simulink model "FSFB"  (R2023a)
settings: Solver=VariableStepAuto  StartTime=0.0  StopTime=60  RelTol=1e-8
values from neighbouring files (symbols this model uses):
  e_0 = [0;0;0]    [as5.m]
  eps_0 = [.2; -.5; .3]    [as5.m]
  eps_c = [-.2; -.4; .2]    [as5.m]
  eta_0 = sqrt(1- eps_0'*eps_0)    [as5.m]
  eta_c = sqrt(1- eps_c'*eps_c)    [as5.m]
  I = [1200 0 0; 0 2000 0; 0 0 2800]    [as5.m]
  k_d = I * eye(3) * 2 * zeta * omega_n    [as5.m]
  k_p = I * eye(3) * 2 * omega_n^2    [as5.m]
  omega_0 = [.1; -.05; .05]    [as5.m]
settings Model: Creator=renob  LastModifiedBy=rbrown

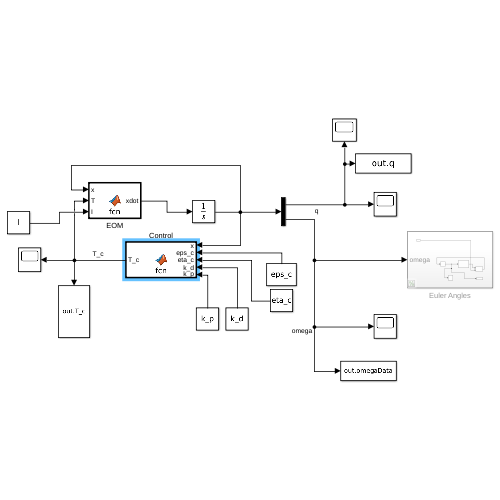
[thumbnail: Simulink's stored preview of the top-level diagram]
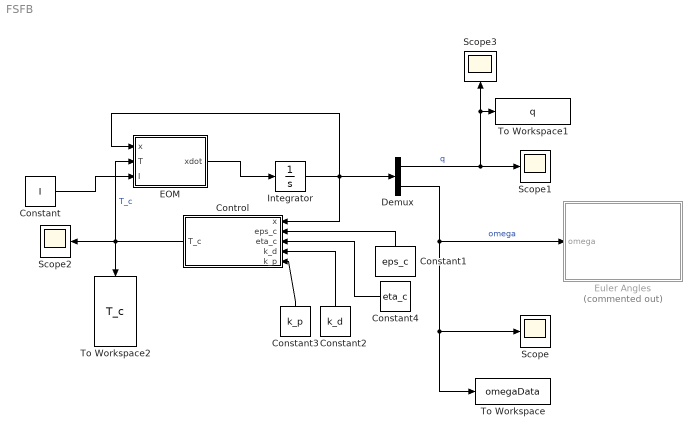
== system FSFB ==
  Constant : Constant  Value=I
  Constant1 : Constant  Value=eps_c
  Constant2 : Constant  Value=k_d
  Constant3 : Constant  Value=k_p  VectorParams1D=off
  Constant4 : Constant  Value=eta_c
  Control : MATLAB Function  TreatAsAtomicUnit=on
  Demux : Demux  Outputs=[-1 3]
  EOM : MATLAB Function  TreatAsAtomicUnit=on
  Euler Angles : Subsystem  Commented=on
  Integrator : Integrator  InitialCondition=[eps_0; eta_0; omega_0]
  Scope{,1..3} (4 alike) : Scope
  To Workspace : ToWorkspace  VariableName=omegaData  SampleTime=-1
  To Workspace1 : ToWorkspace  VariableName=q  SampleTime=-1
  To Workspace2 : ToWorkspace  VariableName=T_c  SampleTime=-1
      settings: Save2DSignal=2-D array (concatenate along first dimension)
  wires:
  Demux/2 -> To Workspace/1, Scope/1, Euler Angles/1(omega)  "omega"
  Demux/1 -> Scope1/1, Scope3/1, To Workspace1/1  "q"
  Constant/1 -> EOM/3(I)
  Integrator/1 -> Control/1(x), EOM/1(x), Demux/1
  EOM/1(xdot) -> Integrator/1
  Control/1(T_c) -> To Workspace2/1, Scope2/1, EOM/2(T)  "T_c"
  Constant1/1 -> Control/2(eps_c)
  Constant2/1 -> Control/4(k_d)
  Constant3/1 -> Control/5(k_p)
  Constant4/1 -> Control/3(eta_c)

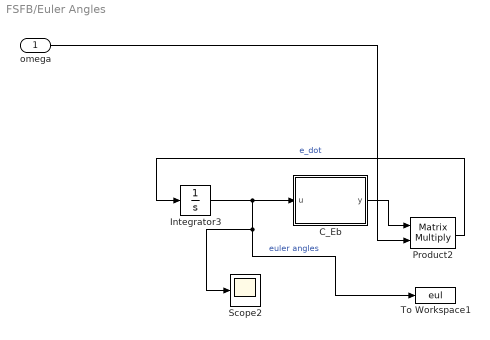
== system FSFB/Euler Angles ==
  omega : Inport
  C_Eb : MATLAB Function  TreatAsAtomicUnit=on
  Integrator3 : Integrator  InitialCondition=e_0
  Product2 : Product  Multiplication=Matrix(*)
  Scope2 : Scope
  To Workspace1 : ToWorkspace  VariableName=eul  SampleTime=-1
  wires:
  Product2/1 -> Integrator3/1  "e_dot"
  C_Eb/1(y) -> Product2/1
  omega/1 -> Product2/2
  Integrator3/1 -> To Workspace1/1, Scope2/1, C_Eb/1(u)  "euler angles"

== matlab function FSFB/Control ==
  data: x input; eps_c input; eta_c input; k_d input; T_c output; k_p input
function T_c = fcn(x, eps_c, eta_c, k_d, k_p)

quat_err = quatmultiply(quatconj([x(4) x(1:3)']), [eta_c eps_c']);
omega = x(5:7);
T_c = -k_p* quat_err(2:4)' -k_d*omega;

== matlab function FSFB/EOM ==
  data: x input; T input; xdot output; I input
function xdot = fcn(x, T, I)

xdot = zeros(7,1);
eps = x(1:3); 
eta = x(4);
omega = x(5:7);
xdot(1:3) = .5 * (eta *eye(3) + xmat(eps)) * omega;
xdot(4) = -.5 * eps' * omega;
xdot(5:7) = I^-1 * (-xmat(omega)*I*omega + T);

end

== matlab function FSFB/Euler Angles/C_Eb ==
  data: u input; y output
function y = fcn(u)

y = C_e(u);
